simulink model "SolarSail"  (R2024a)
settings: Solver=ode3  StartTime=0.0  StopTime=2*24*60*60  FixedStep=30  MinStep=1  RelTol=1e-3
model workspace (MAT data in the model file):
  I_s = [344.15  0  0; 0  344.15  0; 0  0  688.24]
  LocalBodyOffset = [45 0 0]
undefined symbols (not defined in the file): IAU, juliandate, WMM2020
libraries: aerolibutil x15, matrix_library x14, simulink_extras x6, sharedtransform x5, aerolibtransform2 x4, aerolibconvert2 x4, aerolibatmos2 x1, aerolibsatdyn x1, aerolibobsolete x1, aerolibattitudesys x1, simulink x1, vrlib x1
(part 2 of 2)

== system SolarSail/RCDs/RCD4 ==
  Input Signal : Inport
  F_ON : Inport  Port=2
  F_OFF : Inport  Port=3
  Constant : Constant  Value=[0;0]
  Constant1 : Constant  Value=[0;0]
  If : If  IfExpression=u1 == 0  ElseIfExpressions=u1 == 1  ShowElse=off
  If Action Subsystem : Subsystem  TreatAsAtomicUnit=on
  If Action Subsystem1 : Subsystem  TreatAsAtomicUnit=on
  Merge : Merge
  RCD radius : Constant  Value=[0;-2.5;0]
  Vector Concatenate : Concatenate
  Vector Concatenate1 : Concatenate
  torque vector : Outport
  wires:
  Input Signal/1 -> If/1
  If/1 -> If Action Subsystem/Action
  Merge/1 -> torque vector/1
  If Action Subsystem/1(Out1) -> Merge/1
  If/2 -> If Action Subsystem1/Action
  If Action Subsystem1/1(Out1) -> Merge/2
  RCD radius/1 -> If Action Subsystem/2(radius), If Action Subsystem1/2(radius)
  Vector Concatenate/1 -> If Action Subsystem/1(F_OFF)
  Constant/1 -> Vector Concatenate/1
  F_OFF/1 -> Vector Concatenate/2
  F_ON/1 -> Vector Concatenate1/2
  Constant1/1 -> Vector Concatenate1/1
  Vector Concatenate1/1 -> If Action Subsystem1/1(F_ON)

== system SolarSail/RCDs/Specular Force ==
  SRP : Inport
  Area : Inport  Port=2
  SunAngle : Inport  Port=3
  Cos : Trigonometry  Operator=cos
  Product : Product  Inputs=3
  Square : Math  Operator=square
  vector : Gain  Gain=2
  Spec Force : Outport
  wires:
  Product/1 -> vector/1
  SunAngle/1 -> Cos/1
  Cos/1 -> Square/1
  SRP/1 -> Product/1
  Area/1 -> Product/2
  Square/1 -> Product/3
  vector/1 -> Spec Force/1

== system SolarSail/Reaction Wheels/T to w ==
  w_prev : Inport
  T : Inport  Port=2
  I : Inport  Port=3
  dT : Inport  Port=4
  Add : Sum
  Constant : Constant  Value=-1
  Divide : Product  Inputs=*/**
  w : Outport
  wires:
  T/1 -> Divide/1
  I/1 -> Divide/2
  dT/1 -> Divide/3
  Divide/1 -> Add/2
  w_prev/1 -> Add/1
  Add/1 -> w/1
  Constant/1 -> Divide/4

== system SolarSail/Reaction Wheels/deltaT ==
  Clock : Clock
  Constant : Constant  Value=0.01
  Memory : Memory
  Min : MinMax  Function=max  Inputs=2
  Subtract : Sum  Inputs=+-
  dT : Outport
  wires:
  Clock/1 -> Memory/1, Subtract/1
  Memory/1 -> Subtract/2
  Subtract/1 -> Min/1
  Constant/1 -> Min/2
  Min/1 -> dT/1

== system SolarSail/Reaction Wheels/w to T ==
  w_f : Inport
  w_i : Inport  Port=2
  I : Inport  Port=3
  dT : Inport  Port=4
  Constant : Constant  Value=-1
  Divide : Product  Inputs=***/
  Subtract : Sum  Inputs=+-
  T : Outport
  wires:
  Constant/1 -> Divide/1
  I/1 -> Divide/2
  w_i/1 -> Subtract/2
  w_f/1 -> Subtract/1
  Subtract/1 -> Divide/3
  dT/1 -> Divide/4
  Divide/1 -> T/1

== system SolarSail/SRP/Absorption Force ==
  SRP : Inport
  Area : Inport  Port=2
  SunAngle : Inport  Port=3
  S_hat : Inport  Port=4
  C_a : Inport  Port=5
  F_sun : Subsystem
  Product : Product
  Abs Force : Outport
  wires:
  F_sun/1(F_sun) -> Abs Force/1
  SRP/1 -> F_sun/1(SRP)
  SunAngle/1 -> F_sun/3(sun angle)
  Area/1 -> Product/1
  C_a/1 -> Product/2
  Product/1 -> F_sun/2(area)
  S_hat/1 -> F_sun/4(S_hat)

== system SolarSail/SRP/Diffusive Force ==
  SRP : Inport
  Area : Inport  Port=2
  SunAngle : Inport  Port=3
  S_hat : Inport  Port=4
  C_d : Inport  Port=5
  Add : Sum
  F_normal : Subsystem
  F_sun : Subsystem
  Product : Product
  Diff Force : Outport
  wires:
  F_sun/1(F_sun) -> Add/2
  F_normal/1(F_normal) -> Add/1
  Add/1 -> Diff Force/1
  SRP/1 -> F_normal/1(SRP), F_sun/1(SRP)
  SunAngle/1 -> F_sun/3(sun angle), F_normal/3(sun angle)
  Area/1 -> Product/1
  C_d/1 -> Product/2
  Product/1 -> F_sun/2(area), F_normal/2(area)
  S_hat/1 -> F_sun/4(S_hat)

== system SolarSail/SRP/Specular Force ==
  SRP : Inport
  Area : Inport  Port=2
  SunAngle : Inport  Port=3
  C_s : Inport  Port=4
  Cos : Trigonometry  Operator=cos
  Product : Product  Inputs=4
  Product1 : Product
  Square : Math  Operator=square
  unitVector : Subsystem
  vector : Gain  Gain=[0;0;-2]
  Spec Force : Outport
  wires:
  Product/1 -> vector/1
  SunAngle/1 -> Cos/1
  Cos/1 -> Square/1, unitVector/1(X)
  SRP/1 -> Product/1
  Area/1 -> Product/2
  Square/1 -> Product/3
  C_s/1 -> Product/4
  vector/1 -> Product1/1
  unitVector/1(X_hat) -> Product1/2  "Direction"
  Product1/1 -> Spec Force/1

== system SolarSail/Sun Angle/unitVector ==
  X : Inport
  Divide : Product  Inputs=*/
  Dot Product : DotProduct  OutDataTypeStr=Inherit: Inherit via internal rule
  Square Root : Sqrt
  X_hat : Outport
  wires:
  X/1 -> Divide/1, Dot Product/2, Dot Product/1
  Dot Product/1 -> Square Root/1
  Square Root/1 -> Divide/2
  Divide/1 -> X_hat/1

== system SolarSail/icrf2lvlh/DCM_icrf2lvlh ==
  pos : Inport
  vel : Inport  Port=2
  Cross Product : matrix_library/Cross Product
  Cross Product1 : matrix_library/Cross Product
  Vector Concatenate : Concatenate  NumInputs=3  Mode=Multidimensional array  ConcatenateDimension=2
  unitVector : Subsystem
  unitVector1 : Subsystem
  unitVector2 : Subsystem
  DCM : Outport
  wires:
  pos/1 -> Cross Product/1, unitVector/1(X)
  unitVector/1(X_hat) -> Vector Concatenate/1, Cross Product1/2  "X_hat"
  vel/1 -> Cross Product/2
  Cross Product/1 -> unitVector1/1(X)  "h"
  unitVector1/1(X_hat) -> Vector Concatenate/3, Cross Product1/1  "Z_hat"
  Cross Product1/1 -> unitVector2/1(X)  "Y"
  unitVector2/1(X_hat) -> Vector Concatenate/2  "Y_hat"
  Vector Concatenate/1 -> DCM/1

== system SolarSail/Atmospheric Drag/Drag Angle/unitVector ==
  X : Inport
  Divide : Product  Inputs=*/
  Dot Product : DotProduct  OutDataTypeStr=Inherit: Inherit via internal rule
  Square Root : Sqrt
  X_hat : Outport
  wires:
  X/1 -> Divide/1, Dot Product/2, Dot Product/1
  Dot Product/1 -> Square Root/1
  Square Root/1 -> Divide/2
  Divide/1 -> X_hat/1

== system SolarSail/Atmospheric Drag/Drag Angle/unitVector1 ==
  X : Inport
  Divide : Product  Inputs=*/
  Dot Product : DotProduct  OutDataTypeStr=Inherit: Inherit via internal rule
  Square Root : Sqrt
  X_hat : Outport
  wires:
  X/1 -> Divide/1, Dot Product/2, Dot Product/1
  Dot Product/1 -> Square Root/1
  Square Root/1 -> Divide/2
  Divide/1 -> X_hat/1

== system SolarSail/CubeSat Animation/Antenna Position to VRML/ECEF to VRML ==
  M : Inport  PortDimensions=3
  Selector : Selector  InputPortWidth=3  IndexOptions=Index vector (dialog)  Indices=[2 3 1]  OutputSizes=1
  VR : Outport  PortDimensions=3  VectorParamsAs1DForOutWhenUnconnected=off
  wires:
  M/1 -> Selector/1
  Selector/1 -> VR/1

== system SolarSail/CubeSat Animation/Compute Earth Rotation Rate/Quaternion to VRML ==
  q : Inport
  Demux : Demux
  Gain : Gain  Gain=2
  Gain3 : Gain  Gain=[-1 1 1 1]
  Mux : Mux
  Selector : Selector  InputPortWidth=4  IndexOptions=Index vector (dialog)  Indices=[2 4 3 1]  OutputSizes=1
  Trigonometric Function : Trigonometry  Operator=acos
  AxisAngle : Outport  VectorParamsAs1DForOutWhenUnconnected=off
  wires:
  Demux/1 -> Trigonometric Function/1
  Trigonometric Function/1 -> Gain/1
  Mux/1 -> Selector/1
  q/1 -> Demux/1
  Gain3/1 -> AxisAngle/1
  Selector/1 -> Gain3/1
  Gain/1 -> Mux/1
  Demux/2 -> Mux/2
  Demux/3 -> Mux/3
  Demux/4 -> Mux/4

== system SolarSail/CubeSat Animation/Compute Umbra Translation/unitVec ==
  I : Inport
  Divide : Product  Inputs=*/
  Dot Product : DotProduct  OutDataTypeStr=Inherit: Inherit via internal rule
  Sqrt : Sqrt
  O : Outport  VectorParamsAs1DForOutWhenUnconnected=off
  wires:
  Dot Product/1 -> Sqrt/1
  I/1 -> Divide/1, Dot Product/1, Dot Product/2
  Divide/1 -> O/1
  Sqrt/1 -> Divide/2

== system SolarSail/CubeSat Animation/Sat Position to VRML/ECEF to VRML ==
  M : Inport  PortDimensions=3
  Selector : Selector  InputPortWidth=3  IndexOptions=Index vector (dialog)  Indices=[2 3 1]  OutputSizes=1
  VR : Outport  PortDimensions=3  VectorParamsAs1DForOutWhenUnconnected=off
  wires:
  M/1 -> Selector/1
  Selector/1 -> VR/1

== system SolarSail/CubeSat Animation/Sun Position to VRML/ECEF to VRML ==
  M : Inport  PortDimensions=3
  Selector : Selector  InputPortWidth=3  IndexOptions=Index vector (dialog)  Indices=[2 3 1]  OutputSizes=1
  VR : Outport  PortDimensions=3  VectorParamsAs1DForOutWhenUnconnected=off
  wires:
  M/1 -> Selector/1
  Selector/1 -> VR/1

== system SolarSail/RCDs/Absorption Force/F_sun ==
  SRP : Inport
  area : Inport  Port=2
  sun angle : Inport  Port=3
  Abs : Abs  SaturateOnIntegerOverflow=off
  Cos : Trigonometry  Operator=cos
  Product1 : Product  Inputs=3
  F_sun : Outport
  wires:
  Cos/1 -> Abs/1
  sun angle/1 -> Cos/1
  area/1 -> Product1/2  "area"
  SRP/1 -> Product1/1
  Product1/1 -> F_sun/1
  Abs/1 -> Product1/3

== system SolarSail/RCDs/Diffusive Force/F_normal ==
  SRP : Inport
  area : Inport  Port=2
  sun angle : Inport  Port=3
  Cos : Trigonometry  Operator=cos
  Gain : Gain  Gain=2/3
  Product1 : Product  Inputs=3
  F_normal : Outport
  wires:
  Product1/1 -> Gain/1
  SRP/1 -> Product1/1
  area/1 -> Product1/2  "area"
  sun angle/1 -> Cos/1
  Gain/1 -> F_normal/1
  Cos/1 -> Product1/3

== system SolarSail/RCDs/Diffusive Force/F_sun ==
  SRP : Inport
  area : Inport  Port=2
  sun angle : Inport  Port=3
  Abs : Abs  SaturateOnIntegerOverflow=off
  Cos : Trigonometry  Operator=cos
  Product1 : Product  Inputs=3
  F_sun : Outport
  wires:
  Cos/1 -> Abs/1
  sun angle/1 -> Cos/1
  area/1 -> Product1/2  "area"
  SRP/1 -> Product1/1
  Product1/1 -> F_sun/1
  Abs/1 -> Product1/3

== system SolarSail/RCDs/RCD1/If Action Subsystem ==
  F_OFF : Inport
  radius : Inport  Port=2
  Action Port : ActionPort  ActionPortLabel=if(u1 == 0)
  Cross Product : matrix_library/Cross Product
  Out1 : Outport
  wires:
  Cross Product/1 -> Out1/1
  F_OFF/1 -> Cross Product/2
  radius/1 -> Cross Product/1

== system SolarSail/RCDs/RCD1/If Action Subsystem1 ==
  F_ON : Inport
  radius : Inport  Port=2
  Action Port : ActionPort  ActionPortLabel=elseif(u1 == 1)
  Cross Product : matrix_library/Cross Product
  Out1 : Outport
  wires:
  Cross Product/1 -> Out1/1
  F_ON/1 -> Cross Product/2
  radius/1 -> Cross Product/1

== system SolarSail/RCDs/RCD2/If Action Subsystem ==
  F_OFF : Inport
  radius : Inport  Port=2
  Action Port : ActionPort  ActionPortLabel=if(u1 == 0)
  Cross Product : matrix_library/Cross Product
  Out1 : Outport
  wires:
  Cross Product/1 -> Out1/1
  F_OFF/1 -> Cross Product/2
  radius/1 -> Cross Product/1

== system SolarSail/RCDs/RCD2/If Action Subsystem1 ==
  F_ON : Inport
  radius : Inport  Port=2
  Action Port : ActionPort  ActionPortLabel=elseif(u1 == 1)
  Cross Product : matrix_library/Cross Product
  Out1 : Outport
  wires:
  Cross Product/1 -> Out1/1
  F_ON/1 -> Cross Product/2
  radius/1 -> Cross Product/1

== system SolarSail/RCDs/RCD3/If Action Subsystem ==
  F_OFF : Inport
  radius : Inport  Port=2
  Action Port : ActionPort  ActionPortLabel=if(u1 == 0)
  Cross Product : matrix_library/Cross Product
  Out1 : Outport
  wires:
  Cross Product/1 -> Out1/1
  F_OFF/1 -> Cross Product/2
  radius/1 -> Cross Product/1

== system SolarSail/RCDs/RCD3/If Action Subsystem1 ==
  F_ON : Inport
  radius : Inport  Port=2
  Action Port : ActionPort  ActionPortLabel=elseif(u1 == 1)
  Cross Product : matrix_library/Cross Product
  Out1 : Outport
  wires:
  Cross Product/1 -> Out1/1
  F_ON/1 -> Cross Product/2
  radius/1 -> Cross Product/1

== system SolarSail/RCDs/RCD4/If Action Subsystem ==
  F_OFF : Inport
  radius : Inport  Port=2
  Action Port : ActionPort  ActionPortLabel=if(u1 == 0)
  Cross Product : matrix_library/Cross Product
  Out1 : Outport
  wires:
  Cross Product/1 -> Out1/1
  F_OFF/1 -> Cross Product/2
  radius/1 -> Cross Product/1

== system SolarSail/RCDs/RCD4/If Action Subsystem1 ==
  F_ON : Inport
  radius : Inport  Port=2
  Action Port : ActionPort  ActionPortLabel=elseif(u1 == 1)
  Cross Product : matrix_library/Cross Product
  Out1 : Outport
  wires:
  Cross Product/1 -> Out1/1
  F_ON/1 -> Cross Product/2
  radius/1 -> Cross Product/1

== system SolarSail/SRP/Absorption Force/F_sun ==
  SRP : Inport
  area : Inport  Port=2
  sun angle : Inport  Port=3
  S_hat : Inport  Port=4
  Abs : Abs  SaturateOnIntegerOverflow=off
  Cos : Trigonometry  Operator=cos
  Product : Product
  Product1 : Product  Inputs=3
  F_sun : Outport
  wires:
  Cos/1 -> Abs/1
  sun angle/1 -> Cos/1
  area/1 -> Product1/2  "area"
  SRP/1 -> Product1/1
  Product/1 -> F_sun/1
  S_hat/1 -> Product/2
  Product1/1 -> Product/1
  Abs/1 -> Product1/3

== system SolarSail/SRP/Diffusive Force/F_normal ==
  SRP : Inport
  area : Inport  Port=2
  sun angle : Inport  Port=3
  Cos : Trigonometry  Operator=cos
  Gain : Gain  Gain=[0;0;-2/3]
  Product1 : Product  Inputs=3
  F_normal : Outport
  wires:
  Product1/1 -> Gain/1
  SRP/1 -> Product1/1
  area/1 -> Product1/2  "area"
  sun angle/1 -> Cos/1
  Gain/1 -> F_normal/1
  Cos/1 -> Product1/3

== system SolarSail/SRP/Diffusive Force/F_sun ==
  SRP : Inport
  area : Inport  Port=2
  sun angle : Inport  Port=3
  S_hat : Inport  Port=4
  Abs : Abs  SaturateOnIntegerOverflow=off
  Cos : Trigonometry  Operator=cos
  Product : Product
  Product1 : Product  Inputs=3
  F_sun : Outport
  wires:
  Cos/1 -> Abs/1
  sun angle/1 -> Cos/1
  area/1 -> Product1/2  "area"
  SRP/1 -> Product1/1
  Product/1 -> F_sun/1
  S_hat/1 -> Product/2
  Product1/1 -> Product/1
  Abs/1 -> Product1/3

== system SolarSail/SRP/Specular Force/unitVector ==
  X : Inport
  Divide : Product  Inputs=*/
  Dot Product : DotProduct  OutDataTypeStr=Inherit: Inherit via internal rule
  Square Root : Sqrt
  X_hat : Outport
  wires:
  X/1 -> Divide/1, Dot Product/2, Dot Product/1
  Dot Product/1 -> Square Root/1
  Square Root/1 -> Divide/2
  Divide/1 -> X_hat/1

== system SolarSail/icrf2lvlh/DCM_icrf2lvlh/unitVector ==
  X : Inport
  Divide : Product  Inputs=*/
  Dot Product : DotProduct  OutDataTypeStr=Inherit: Inherit via internal rule
  Square Root : Sqrt
  X_hat : Outport
  wires:
  X/1 -> Divide/1, Dot Product/2, Dot Product/1
  Dot Product/1 -> Square Root/1
  Square Root/1 -> Divide/2
  Divide/1 -> X_hat/1

== system SolarSail/icrf2lvlh/DCM_icrf2lvlh/unitVector1 ==
  X : Inport
  Divide : Product  Inputs=*/
  Dot Product : DotProduct  OutDataTypeStr=Inherit: Inherit via internal rule
  Square Root : Sqrt
  X_hat : Outport
  wires:
  X/1 -> Divide/1, Dot Product/2, Dot Product/1
  Dot Product/1 -> Square Root/1
  Square Root/1 -> Divide/2
  Divide/1 -> X_hat/1

== system SolarSail/icrf2lvlh/DCM_icrf2lvlh/unitVector2 ==
  X : Inport
  Divide : Product  Inputs=*/
  Dot Product : DotProduct  OutDataTypeStr=Inherit: Inherit via internal rule
  Square Root : Sqrt
  X_hat : Outport
  wires:
  X/1 -> Divide/1, Dot Product/2, Dot Product/1
  Dot Product/1 -> Square Root/1
  Square Root/1 -> Divide/2
  Divide/1 -> X_hat/1

== matlab function SolarSail/SetMode/MATLAB Function ==
  data: Mode output; w input; w_on input; w_off input; reset output
function [Mode,reset] = setMode(w, w_on, w_off)

% Mode is 0 or 1 (EO or Sun)
if ((w(1) > w_on || w(1) < -w_on) || (w(2) > w_on || w(2) < -w_on))
    % Set Sun-pointing Mode (1)
    Mode = true;
    reset = false;
elseif ((w(1) < w_off && w(1) > -w_off) && (w(2) < w_off && w(2) > -w_off))
    % Set Earth Observation Mode (0)
    Mode = false;
    reset = true;
else
    % Keep same state
    Mode = false;
    reset = false;
end

== matlab function SolarSail/IJK2Keplerian/MATLAB Function ==
  data: r_ijk input; a output; v_ijk input; ecc output; incl output; RAAN output; argp output; nu output
function [a,ecc,incl,RAAN,argp,nu] = fcn(r_ijk, v_ijk)

[a,ecc,incl,RAAN,argp,nu] = deal(0.0,0.0,0.0,0.0,0.0,0.0);

% Declare the ijk2keplerian function as extrinsic to prevent code generation
coder.extrinsic('ijk2keplerian');

[a,ecc,incl,RAAN,argp,nu,~,~,~] = ijk2keplerian(r_ijk, v_ijk);

== matlab function SolarSail/Unwrap Angles ==
  data: angle input; unwrapped output
function unwrapped = unwrapAngle(angle)
% This function unwraps the input angle (in degrees) for a 3x1 vector input.
% It assumes a sample-based input where 'angle' is the current measurement vector.
%
% The function uses persistent variables to store the previous angle and the
% cumulative offset for each element.

persistent prevAngle offset

if isempty(prevAngle)
    % Initialize on the first call with the same size as the input angle vector.
    prevAngle = angle;
    offset = zeros(size(angle));
end

% Compute the difference between current and previous angles for each element.
delta = angle - prevAngle;

% Process each element to detect and adjust for wrapping.
for i = 1:length(angle)
    if delta(i) > pi
        offset(i) = offset(i) - 2*pi;
    elseif delta(i) < -pi
        offset(i) = offset(i) + 2*pi;
    end
end

% Apply the cumulative offset.
unwrapped = angle + offset;

% Update the previous angle for the next sample.
prevAngle = angle;

== matlab function SolarSail/RCD Controller/MATLAB Function ==
  data: RCD2 output; reset2 output; RCD4 output; w_x input; w_on input; w_off input; reset4 output; SunAngle input; Mode input
function [RCD2, reset2, RCD4, reset4] = fcn(w_x, w_on, w_off, SunAngle, Mode)
% Check if SunAngle within operating range (i.e. F_spec > F_diff)
if (SunAngle < 0.84 && SunAngle > -0.84 && Mode == 1)
    if (-w_x > w_on)
        % Turn one side on (negative torque)
        RCD2 = true;
        RCD4 = false;
        reset2 = false;
        reset4 = true;
    elseif (-w_x < -w_on)
        % Turn other side on (positive torque)
        RCD2 = false;
        RCD4 = true;
        reset2 = true;
        reset4 = false;
    elseif (-w_x < w_off && -w_x > -w_off)
        % Turn both off
        RCD2 = false;
        RCD4 = false;
        reset2 = true;
        reset4 = true;
    else
        % Keep same state
        RCD2 = false;
        RCD4 = false;
        reset2 = false;
        reset4 = false;
    end
else
    % Turn both off
    RCD2 = false;
    RCD4 = false;
    reset2 = true;
    reset4 = true;
end

== matlab function SolarSail/RCD Controller/MATLAB Function1 ==
  data: RCD1 output; reset1 output; RCD3 output; w_y input; w_on input; w_off input; reset3 output; SunAngle input; Mode input
function [RCD1, reset1, RCD3, reset3] = fcn(w_y, w_on, w_off, SunAngle, Mode)
% Check if SunAngle within operating range (i.e. F_spec > F_diff)
if (SunAngle < 0.84 && SunAngle > -0.84 && Mode == 1)
    if (-w_y > w_on)
        % Turn one side on (negative torque)
        RCD1 = false;
        RCD3 = true;
        reset1 = true;
        reset3 = false;
    elseif (-w_y < -w_on)
        % Turn other side on (positive torque)
        RCD1 = true;
        RCD3 = false;
        reset1 = false;
        reset3 = true;
    elseif (-w_y < w_off && -w_y > -w_off)
        % Turn both off
        RCD1 = false;
        RCD3 = false;
        reset1 = true;
        reset3 = true;
    else
        % Keep same state
        RCD1 = false;
        RCD3 = false;
        reset1 = false;
        reset3 = false;
    end
else
    % Turn both off
    RCD1 = false;
    RCD3 = false;
    reset1 = true;
    reset3 = true;
end
